simulink model "buck_boost_forcebuck_openloop"  (R2023b)
settings: Solver=VariableStepAuto  StartTime=0.0  StopTime=0.05  RelTol=1e-3
libraries: spsSeriesRLCBranchLib x5, spsMosfetLib x4, spsCurrentMeasurementLib x1, spsDCVoltageSourceLib x1, simulink x1, spsVoltageMeasurementLib x1, sps_lib x1
settings Model: Creator=sch  LastModifiedBy=sch

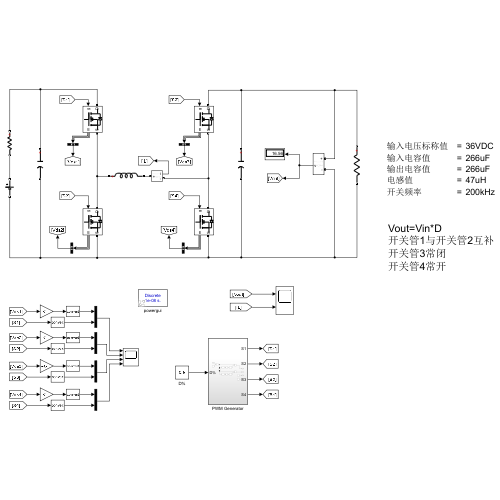
[thumbnail: Simulink's stored preview of the top-level diagram]
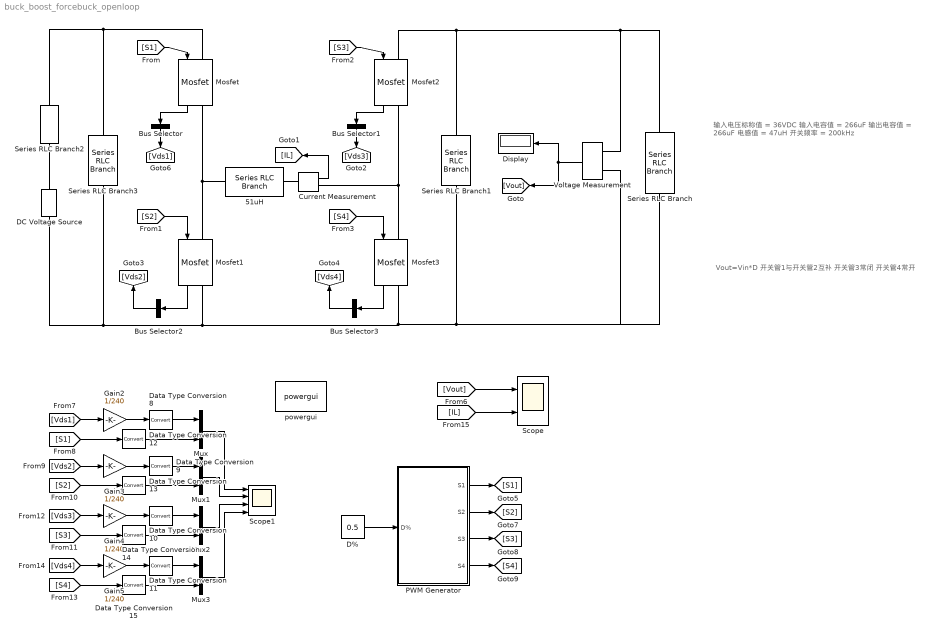
== system buck_boost_forcebuck_openloop ==
  note: Vout=Vin*D
      | 开关管1与开关管2互补
      | 开关管3常闭
      | 开关管4常开
  note: 输入电压标称值 = 36VDC
      | 输入电容值 = 266uF
      | 输出电容值 = 266uF
      | 电感值 = 47uH
      | 开关频率 = 200kHz
  51uH : spsSeriesRLCBranchLib/Series RLC Branch  LConnTagsString=__new0  RConnTagsString=__new0  BranchType=L  Resistance=1  Inductance=47e-6  SetiL0=off  InitialCurrent=0  Capacitance=1e-6  Setx0=off  InitialVoltage=0  Measurements=Branch current
  Bus Selector{,1..3} (4 alike) : BusSelector  OutputSignals=MOSFET voltage  OutputAsBus=on
  Current Measurement : spsCurrentMeasurementLib/Current Measurement  PhasorSimulation=off  OutputType=Complex  PSBequivalent=0
  D% : Constant  Value=0.5
  DC Voltage Source : spsDCVoltageSourceLib/DC Voltage Source  Amplitude=36  Measurements=None
  Data Type Conversion{8..15} (8 alike) : DataTypeConversion  SaturateOnIntegerOverflow=off  RndMeth=Floor
  Display : Display
  Gain{2..5} (4 alike) : Gain  Gain=1/240
  Mosfet{,1..3} (4 alike) : spsMosfetLib/Mosfet  Ron=0.0063  Lon=0  Rd=0.001  Vfd=0  IC=0  Rs=1e5  Cs=inf  Measurements=on
  Mux{,1..3} (4 alike) : Mux  Inputs=2
  PWM Generator : Subsystem
  Scope : Scope  NumInputPorts=2
  Scope1 : Scope  NumInputPorts=4
  Series RLC Branch : spsSeriesRLCBranchLib/Series RLC Branch  LConnTagsString=__new0  RConnTagsString=__new0  BranchType=R  Resistance=5  Inductance=1e-3  SetiL0=off  InitialCurrent=0  Capacitance=1e-6  Setx0=off  InitialVoltage=0  Measurements=None
  Series RLC Branch1 : spsSeriesRLCBranchLib/Series RLC Branch  LConnTagsString=__new0  RConnTagsString=__new0  BranchType=C  Resistance=1  Inductance=5.6e-6  SetiL0=off  InitialCurrent=0  Capacitance=266e-6  Setx0=off  InitialVoltage=0  Measurements=None
  Series RLC Branch2 : spsSeriesRLCBranchLib/Series RLC Branch  LConnTagsString=__new0  RConnTagsString=__new0  BranchType=R  Resistance=1e-3  Inductance=1e-3  SetiL0=off  InitialCurrent=0  Capacitance=1e-6  Setx0=off  InitialVoltage=0  Measurements=None
  Series RLC Branch3 : spsSeriesRLCBranchLib/Series RLC Branch  LConnTagsString=__new0  RConnTagsString=__new0  BranchType=C  Resistance=1  Inductance=5.6e-6  SetiL0=off  InitialCurrent=0  Capacitance=266e-6  Setx0=on  InitialVoltage=36  Measurements=None
  Voltage Measurement : spsVoltageMeasurementLib/Voltage Measurement  PhasorSimulation=off  OutputType=Complex  PSBequivalent=0
  powergui : sps_lib/powergui  Priority=1  SimulationMode=Discrete  SampleTime=1e-8  frequency=60  Iterations=50  frequencyindice=0  Pbase=100e6  ErrMax=1e-4  UnitsV=kV  UnitsW=MW  buscounter=0  FunctionMessages=off  echomessages=off  EnableUseOfTLC=off  CurrentSourceSwitches=off  DisableSnubberDevices=off  DisableRonSwitches=off  DisableVfSwitches=off  DisplayEquations=off  AutomaticDiscreteSolvers=off  SolverType=Tustin/Backward Euler (TBE)  Interpol=off  ExternalGateDelay=off  methode=off  Ts=10  x0status=blocks  SPID=off  SwTol=0  HookPort=off  NonlinearTolerance=0  nMaxIteration=15  ContinueOnMaxIteration=off  RestoreLinks=warning  ResistiveCurrentMeasurement=off  Frange=[0:2:500]  Ylog=off  Xlog=on  ShowGrid=off  save=off  variable=ZData  structure=0  ZoomFFT=off  StartTime=0.0  cycles=1  DisplayStyle=1  fundamental=60  FreqAxis=off  MaxFrequency=1000  frequencyindicesteady=1  RmsSteady=1  display=off
  wires:
  Voltage Measurement/1 -> [Vout], Display/1
  Gain3/1 -> Data Type Conversion9/1
  Data Type Conversion12/1 -> Mux/2
  Gain5/1 -> Data Type Conversion11/1
  PWM Generator/2(S2) -> [S2]
  [Vout] -> Scope/1
  Current Measurement/1 -> [IL]
  PWM Generator/1(S1) -> [S1]
  [S2] -> Data Type Conversion13/1
  [IL] -> Scope/2
  Mux3/1 -> Scope1/4
  Bus Selector2/1 -> [Vds2]
  Mux1/1 -> Scope1/2
  [S1] -> Mosfet/1
  Mux/1 -> Scope1/1
  Data Type Conversion11/1 -> Mux3/1
  Bus Selector1/1 -> [Vds3]
  Mosfet1/1 -> Bus Selector2/1
  Data Type Conversion10/1 -> Mux2/1
  [S4] -> Mosfet3/1
  Mosfet/1 -> Bus Selector/1
  [S1] -> Data Type Conversion12/1
  Mosfet3/1 -> Bus Selector3/1
  Gain4/1 -> Data Type Conversion10/1
  [Vds3] -> Gain4/1
  Mosfet2/1 -> Bus Selector1/1
  [S3] -> Mosfet2/1
  Data Type Conversion14/1 -> Mux2/2
  Mux2/1 -> Scope1/3
  [S2] -> Mosfet1/1
  Bus Selector/1 -> [Vds1]
  Gain2/1 -> Data Type Conversion8/1
  Data Type Conversion15/1 -> Mux3/2
  [Vds1] -> Gain2/1
  Data Type Conversion8/1 -> Mux/1
  [Vds4] -> Gain5/1
  [Vds2] -> Gain3/1
  [S3] -> Data Type Conversion14/1
  D%/1 -> PWM Generator/1(D%)
  Data Type Conversion13/1 -> Mux1/2
  PWM Generator/4(S4) -> [S4]
  PWM Generator/3(S3) -> [S3]
  Bus Selector3/1 -> [Vds4]
  Data Type Conversion9/1 -> Mux1/1
  [S4] -> Data Type Conversion15/1
  connections:
  Series RLC Branch1/RConn1 -- Series RLC Branch/RConn1 -- Voltage Measurement/LConn2 -- Mosfet3/RConn1 -- Series RLC Branch3/RConn1 -- DC Voltage Source/LConn1 -- Mosfet1/RConn1
  Series RLC Branch2/LConn1 -- Series RLC Branch3/LConn1 -- Mosfet/LConn1
  Voltage Measurement/LConn1 -- Series RLC Branch/LConn1 -- Series RLC Branch1/LConn1 -- Mosfet2/LConn1
  Mosfet3/LConn1 -- Current Measurement/RConn1 -- Mosfet2/RConn1
  Mosfet1/LConn1 -- 51uH/LConn1 -- Mosfet/RConn1
  DC Voltage Source/RConn1 -- Series RLC Branch2/RConn1
  51uH/RConn1 -- Current Measurement/LConn1

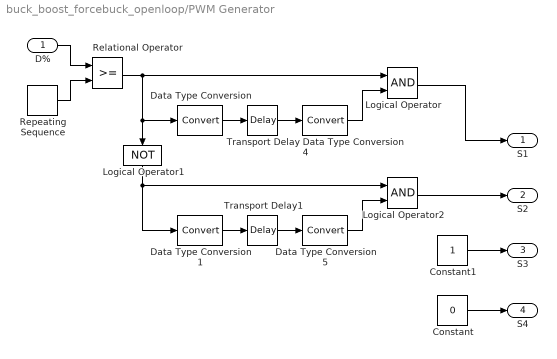
== system buck_boost_forcebuck_openloop/PWM Generator ==
  D% : Inport
  Constant : Constant  Value=0
  Constant1 : Constant
  Data Type Conversion{,1,4..5} (4 alike) : DataTypeConversion  SaturateOnIntegerOverflow=off  RndMeth=Floor
  Logical Operator : Logic  AllPortsSameDT=off  OutDataTypeStr=boolean
  Logical Operator1 : Logic  Operator=NOT  AllPortsSameDT=off  OutDataTypeStr=boolean
  Logical Operator2 : Logic  AllPortsSameDT=off  OutDataTypeStr=boolean
  Relational Operator : RelationalOperator  OutDataTypeStr=boolean  InputSameDT=off
  Repeating Sequence : simulink/Sources/Repeating Sequence  rep_seq_t=[0 0.5/200000 1/200000]  rep_seq_y=[0 1 0]
  Transport Delay : TransportDelay  DelayTime=200e-9
  Transport Delay1 : TransportDelay  DelayTime=200e-9
  S1 : Outport
  S2 : Outport  Port=2
  S3 : Outport  Port=3
  S4 : Outport  Port=4
  wires:
  D%/1 -> Relational Operator/1
  Repeating Sequence/1 -> Relational Operator/2
  Data Type Conversion/1 -> Transport Delay/1
  Data Type Conversion1/1 -> Transport Delay1/1
  Data Type Conversion5/1 -> Logical Operator2/2
  Data Type Conversion4/1 -> Logical Operator/2
  Relational Operator/1 -> Logical Operator/1, Data Type Conversion/1, Logical Operator1/1
  Logical Operator1/1 -> Data Type Conversion1/1, Logical Operator2/1
  Transport Delay1/1 -> Data Type Conversion5/1
  Transport Delay/1 -> Data Type Conversion4/1
  Constant1/1 -> S3/1
  Constant/1 -> S4/1
  Logical Operator/1 -> S1/1
  Logical Operator2/1 -> S2/1
